simulink model "diff_drive_robot_pid_system"  (R2025a)
settings: Solver=ode15s  StartTime=0.0  StopTime=60  MaxStep=0.01  RelTol=1e-4  AbsTol=1e-6
model workspace (MAT data in the model file):
  R_robot = 0.25
  d0 = 1
  k_drag = 0.15
  m = 5
libraries: slpidlib x1
settings Model: Creator=wzy  LastModifiedBy=wzy
settings SolverCC: ZeroCrossAlgorithm=Adaptive

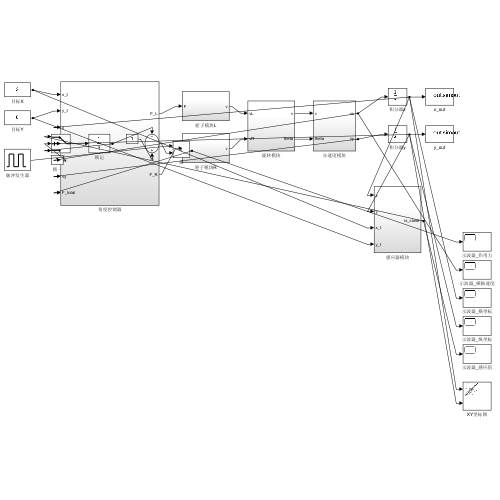
[thumbnail: Simulink's stored preview of the top-level diagram]
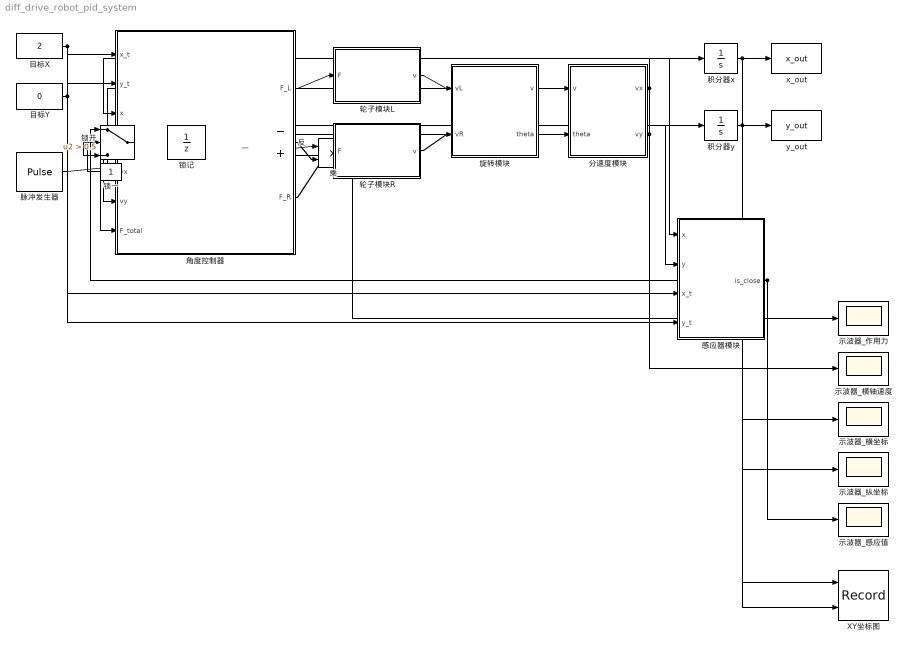
== system diff_drive_robot_pid_system ==
  XY坐标图 : Record  NumPorts=2.0  FileSettingsInternal="{\"entries\":[{\"content\":{\"excelSettings\":{\"content\":{},\"type\":\"Streamout.ExcelSettings\"},\"parquetSettings\":{\"content\":{},\"type\":\"Streamout.ParquetSettings\"}},\"type\":\"Streamout.FileSettingStorage\",\"uuid\":\"\"}],\"packageUris\":[\"http:\\/\\/schema.mathworks.com\\/mf0\\/streamout_blocks\\/R2020a\"],\"version\":\"1.0\"}"  FrameSettings=[0, 0]  Layout=[1 1]  SignalsInternal="{\"entries\":[{\"content\":{\"signals\":[{\"content\":{\"blockPath\":[],\"dimensions\":[1],\"domain\":\"\",\"lineColor\":\"#a2142f\",\"plots\":[ 1 ],\"port\":1,\"signalID\":1,\"signalName\":\"XY Graph:1\"},\"type\":\"RecordBlkView.Signal\",\"uuid\":\"\"},{\"content\":{\"blockPath\":[],\"dimensions\":[1],\"domain\":\"\",\"lineColor\":\"#139fff\",\"plots\":[ 1 ],\"port\":2,\"signalID\":2,\"signalName\":\"XY Graph:2\"},\"type\":\"RecordBlkView.Signal\",\"uuid\":\"\"}]},\"type\":\"RecordBlkView.InputSignals\",\"uuid\":\"\"}],\"packageUris\":[\"http:\\/\\/schema.mathworks.com\\/mf0\\/streamout_blocks\\/R2020a\"],\"version\":\"1.0\"}"  VisualizationBindings="{\"xyplotplugin\":{\"info\":[{\"series\":[{\"bindingParametersList\":[{\"parameter\":\"X-Axis\",\"signalID\":1,\"signalName\":\"XY Graph:1\"},{\"parameter\":\"Y-Axis\",\"signalID\":2,\"signalName\":\"XY Graph:2\"}],\"seriesID\":0}],\"subplotID\":1}]}}"  CompatibilityTag=XY
  x_out : ToWorkspace  VariableName=x_out  SampleTime=-1
  y_out : ToWorkspace  VariableName=y_out  SampleTime=-1
  一 : Constant
  乘 : Product
  分速度模块 : Subsystem
  反 : Sum  Inputs=-+
  感应器模块 : Subsystem
  旋转模块 : Subsystem
  目标X : Constant  Value=2
  目标Y : Constant  Value=0
  示波器_作用力 : Scope
  示波器_感应值 : Scope
  示波器_横坐标 : Scope
  示波器_横轴速度 : Scope
  示波器_纵坐标 : Scope
  积分器x : Integrator
  积分器y : Integrator
  脉冲发生器 : DiscretePulseGenerator  PulseType=Time based  Amplitude=0.8  PulseWidth=0.5
  角度控制器 : Subsystem
  轮子模块L : Subsystem
  轮子模块R : Subsystem
  锁一 : Constant
  锁开 : Switch  Criteria=u2 > Threshold  Threshold=0.5  SaturateOnIntegerOverflow=off  InputSameDT=off
  锁记 : UnitDelay  SampleTime=0.01  HasFrameUpgradeWarning=on
  wires:
  目标X/1 -> 角度控制器/1(x_t), 感应器模块/3(x_t)
  目标Y/1 -> 角度控制器/2(y_t), 感应器模块/4(y_t)
  角度控制器/1(F_L) -> 轮子模块L/1(F)
  角度控制器/2(F_R) -> 轮子模块R/1(F)
  轮子模块L/1(v) -> 旋转模块/1(vL)
  轮子模块R/1(v) -> 旋转模块/2(vR)
  旋转模块/1(v) -> 分速度模块/1(v)
  旋转模块/2(theta) -> 分速度模块/2(theta)
  分速度模块/1(vx) -> 积分器x/1, 角度控制器/5(vx), 示波器_横轴速度/1
  分速度模块/2(vy) -> 积分器y/1, 角度控制器/6(vy)
  积分器x/1 -> 角度控制器/3(x), 感应器模块/1(x), 示波器_横坐标/1, XY坐标图/1, x_out/1
  积分器y/1 -> 角度控制器/4(y), 感应器模块/2(y), 示波器_纵坐标/1, XY坐标图/2, y_out/1
  感应器模块/1(is_close) -> 锁开/1, 示波器_感应值/1
  锁一/1 -> 锁开/2
  锁记/1 -> 锁开/3, 反/1
  锁开/1 -> 锁记/1
  一/1 -> 反/2
  脉冲发生器/1 -> 乘/1
  反/1 -> 乘/2
  乘/1 -> 角度控制器/7(F_total), 示波器_作用力/1

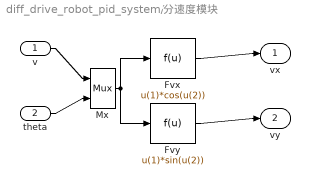
== system diff_drive_robot_pid_system/分速度模块 ==
  v : Inport
  theta : Inport  Port=2
  Fvx : Fcn  Expr=u(1)*cos(u(2))
  Fvy : Fcn  Expr=u(1)*sin(u(2))
  Mx : Mux  Inputs=2
  vx : Outport
  vy : Outport  Port=2
  wires:
  v/1 -> Mx/1
  theta/1 -> Mx/2
  Mx/1 -> Fvx/1, Fvy/1
  Fvx/1 -> vx/1
  Fvy/1 -> vy/1

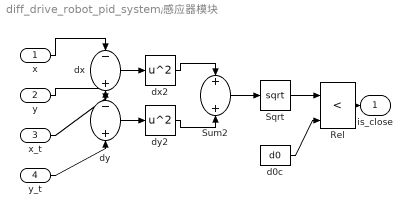
== system diff_drive_robot_pid_system/感应器模块 ==
  x : Inport
  y : Inport  Port=2
  x_t : Inport  Port=3
  y_t : Inport  Port=4
  Rel : RelationalOperator  Operator=<  OutDataTypeStr=boolean  RndMeth=Simplest  InputSameDT=off
  Sqrt : Sqrt
  Sum2 : Sum
  d0c : Constant  Value=d0
  dx : Sum  Inputs=-+
  dx2 : Math  Operator=square
  dy : Sum  Inputs=-+
  dy2 : Math  Operator=square
  is_close : Outport
  wires:
  x/1 -> dx/1
  x_t/1 -> dx/2
  y/1 -> dy/1
  y_t/1 -> dy/2
  dx/1 -> dx2/1
  dy/1 -> dy2/1
  dx2/1 -> Sum2/1
  dy2/1 -> Sum2/2
  Sum2/1 -> Sqrt/1
  Sqrt/1 -> Rel/1
  d0c/1 -> Rel/2
  Rel/1 -> is_close/1

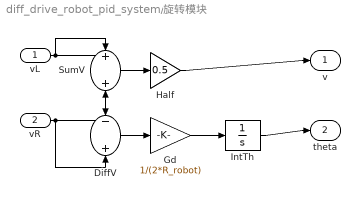
== system diff_drive_robot_pid_system/旋转模块 ==
  vL : Inport
  vR : Inport  Port=2
  DiffV : Sum  Inputs=-+
  Gd : Gain  Gain=1/(2*R_robot)
  Half : Gain  Gain=0.5
  IntTh : Integrator
  SumV : Sum
  v : Outport
  theta : Outport  Port=2
  wires:
  vL/1 -> SumV/1, DiffV/1
  vR/1 -> SumV/2, DiffV/2
  SumV/1 -> Half/1
  Half/1 -> v/1
  DiffV/1 -> Gd/1
  Gd/1 -> IntTh/1
  IntTh/1 -> theta/1

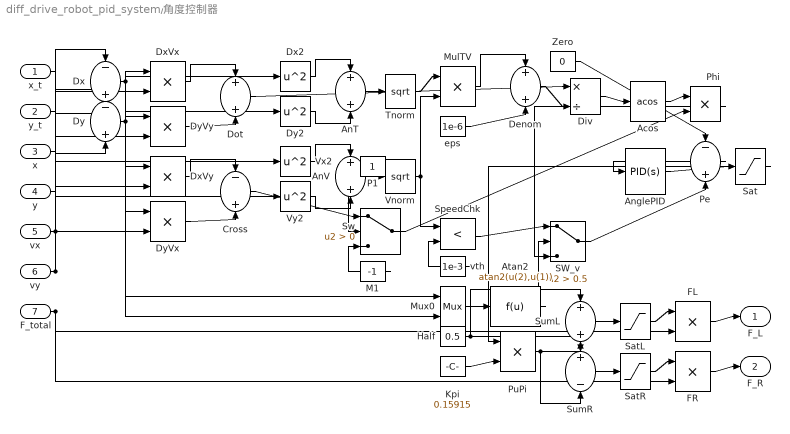
== system diff_drive_robot_pid_system/角度控制器 ==
  x_t : Inport
  y_t : Inport  Port=2
  x : Inport  Port=3
  y : Inport  Port=4
  vx : Inport  Port=5
  vy : Inport  Port=6
  F_total : Inport  Port=7
  Acos : Trigonometry  Operator=acos
  AnT : Sum
  AnV : Sum
  AnglePID : slpidlib/PID Controller  Controller=PID  Form=Parallel  TimeDomain=Continuous-time  UseExternalTs=off  SampleTime=-1  IntegratorMethod=Forward Euler  FilterMethod=Forward Euler  ControllerParametersSource=internal  P=3  I=0  UseKiTs=off  D=0  UseExternalDerivativeSource=off  N=100  UseFilter=on  TunerSelectOption=Transfer Function Based (PID Tuner App)  InitialConditionSource=internal  InitialConditionForIntegrator=0  InitialConditionForFilter=0  DifferentiatorICPrevScaledInput=0  ExternalReset=none  TrackingMode=off  Kt=1  LimitOutput=off  SatLimitsSource=internal  UpperSaturationLimit=inf  LowerSaturationLimit=-inf  LinearizeAsGain=on  AntiWindupMode=none  Kb=1  LimitIntegrator=off  UpperIntegratorSaturationLimit=inf  LowerIntegratorSaturationLimit=-inf  POutMin=[]  POutMax=[]  IOutMin=[]  IOutMax=[]  DOutMin=[]  DOutMax=[]  NOutMin=[]  NOutMax=[]  SumOutMin=[]  SumOutMax=[]  SaturationOutMin=[]  SaturationOutMax=[]  PParamMin=[]  PParamMax=[]  IParamMin=[]  IParamMax=[]  DParamMin=[]  DParamMax=[]  NParamMin=[]  NParamMax=[]  KbParamMin=[]  KbParamMax=[]  KtParamMin=[]  KtParamMax=[]  KbOutMin=[]  KbOutMax=[]  KtOutMin=[]  KtOutMax=[]  IntegratorOutMin=[]  IntegratorOutMax=[]  FilterOutMin=[]  FilterOutMax=[]  SumI1OutMin=[]  SumI1OutMax=[]  SumI2OutMin=[]  SumI2OutMax=[]  SumI3OutMin=[]  SumI3OutMax=[]  SumI4OutMin=[]  SumI4OutMax=[]  SumDOutMin=[]  SumDOutMax=[]  DifferentiatorOutMin=[]  DifferentiatorOutMax=[]  FilterDiffOutCoefMin=[]  FilterDiffOutCoefMax=[]  ReciprocalOutMin=[]  ReciprocalOutMax=[]  SumDenOutMin=[]  SumDenOutMax=[]  SumNumOutMin=[]  SumNumOutMax=[]  DivideOutMin=[]  DivideOutMax=[]  UdiffTsProdOutMin=[]  UdiffTsProdOutMax=[]  NTsProdOutMin=[]  NTsProdOutMax=[]  UintegralTsProdOutMin=[]  UintegralTsProdOutMax=[]  UngainTsProdOutMin=[]  UngainTsProdOutMax=[]  ClampingZeroOutDataTypeStr=Inherit: Inherit via back propagation  ClampingZeroOutMin=[]  ClampingZeroOutMax=[]  FilterDenConstantOutDataTypeStr=Inherit: Inherit via back propagation  FilterDenConstantOutMin=[]  FilterDenConstantOutMax=[]  PCopyOutDataTypeStr=Inherit: Inherit via back propagation  PCopyOutMin=[]  PCopyOutMax=[]  NCopyOutDataTypeStr=Inherit: Inherit via back propagation  NCopyOutMin=[]  NCopyOutMax=[]  IntegratorContinuousStateAttributes=''  IntegratorStateMustResolveToSignalObject=off  IntegratorRTWStateStorageClass=Auto  FilterContinuousStateAttributes=''  FilterStateMustResolveToSignalObject=off  FilterRTWStateStorageClass=Auto  ParallelPVariant=InternalParameters  IdealPVariant=Disabled  IVariant=InternalParameters  DVariant=InternalParameters  IntegratorVariant=Continuous  SatVariant=Disabled  AWVariant=Passthrough  PCopyVariant=Disabled  TRVariant=Disabled  FdbkBlocksVariant=Forward  IdealPFdbkVariant=Disabled  SatFdbkVariant=Disabled  DerivativeFilterVariant=ContFilter  NVariant=InternalParameters  NCopyVariant=Disabled  FilterICVariant=InternalICsFilter  IntegratorICVariant=InternalICs  ExternalResetVariant=Disabled  TRSumVariant=Passthrough  SumFdbkVariant=Disabled  SumVariant=Sum_PID  TsampFilterVariant=InternalTs  TsampNgainVariant=Passthrough  TsampIntegralVariant=Disabled_SignalSpec  ExternalSaturationOutDataTypeStr=Inherit: Same as second input  DerivativeSourceVariant=ErrorSignal  PreIntVariant=InternalPreInt
  Atan2 : Fcn  Expr=atan2(u(2),u(1))
  Cross : Sum  Inputs=-+
  Denom : Sum
  Div : Product  Inputs=*/
  Dot : Sum
  Dx : Sum  Inputs=-+
  Dx2 : Math  Operator=square
  DxVx : Product
  DxVy : Product
  Dy : Sum  Inputs=-+
  Dy2 : Math  Operator=square
  DyVx : Product
  DyVy : Product
  FL : Product
  FR : Product
  Half : Constant  Value=0.5
  Kpi : Constant  Value=0.15915
  M1 : Constant  Value=-1
  MulTV : Product
  Mux0 : Mux  Inputs=2
  P1 : Constant
  Pe : Sum  Inputs=-+
  Phi : Product
  PuPi : Product
  SW_v : Switch  Criteria=u2 > Threshold  Threshold=0.5  ZeroCross=off  SaturateOnIntegerOverflow=off  InputSameDT=off
  Sat : Saturate  UpperLimit=3.1416  LowerLimit=-3.1416  ZeroCross=off
  SatL : Saturate  UpperLimit=1  LowerLimit=-1  ZeroCross=off
  SatR : Saturate  UpperLimit=1  LowerLimit=-1  ZeroCross=off
  SpeedChk : RelationalOperator  Operator=<  OutDataTypeStr=boolean  ZeroCross=off  RndMeth=Simplest  InputSameDT=off
  SumL : Sum
  SumR : Sum  Inputs=+-
  Sw : Switch  Criteria=u2 > Threshold  ZeroCross=off  SaturateOnIntegerOverflow=off  InputSameDT=off
  Tnorm : Sqrt
  Vnorm : Sqrt
  Vx2 : Math  Operator=square
  Vy2 : Math  Operator=square
  Zero : Constant  Value=0
  eps : Constant  Value=1e-6
  vth : Constant  Value=1e-3
  F_L : Outport
  F_R : Outport  Port=2
  wires:
  x/1 -> Dx/1
  x_t/1 -> Dx/2
  y/1 -> Dy/1
  y_t/1 -> Dy/2
  Dx/1 -> DxVx/1, DxVy/1, Dx2/1, Mux0/1
  vx/1 -> DxVx/2, DyVx/2, Vx2/1
  Dy/1 -> DyVy/1, DyVx/1, Dy2/1, Mux0/2
  vy/1 -> DyVy/2, DxVy/2, Vy2/1
  DxVx/1 -> Dot/1
  DyVy/1 -> Dot/2
  DxVy/1 -> Cross/1
  DyVx/1 -> Cross/2
  Dx2/1 -> AnT/1
  Dy2/1 -> AnT/2
  AnT/1 -> Tnorm/1
  Vx2/1 -> AnV/1
  Vy2/1 -> AnV/2
  AnV/1 -> Vnorm/1
  Tnorm/1 -> MulTV/1
  Vnorm/1 -> MulTV/2, SpeedChk/1
  MulTV/1 -> Denom/1
  eps/1 -> Denom/2
  Denom/1 -> Div/2
  Dot/1 -> Div/1
  Div/1 -> Acos/1
  Cross/1 -> Sw/1
  P1/1 -> Sw/2
  M1/1 -> Sw/3
  Acos/1 -> Phi/1
  Sw/1 -> Phi/2
  vth/1 -> SpeedChk/2
  Mux0/1 -> Atan2/1
  SpeedChk/1 -> SW_v/1
  Atan2/1 -> SW_v/2
  Phi/1 -> SW_v/3
  Zero/1 -> Pe/1
  SW_v/1 -> Pe/2
  Pe/1 -> AnglePID/1
  AnglePID/1 -> Sat/1
  Sat/1 -> PuPi/1
  Kpi/1 -> PuPi/2
  Half/1 -> SumL/1, SumR/1
  PuPi/1 -> SumL/2, SumR/2
  SumL/1 -> SatL/1
  SumR/1 -> SatR/1
  SatL/1 -> FL/1
  F_total/1 -> FL/2, FR/2
  SatR/1 -> FR/1
  FL/1 -> F_L/1
  FR/1 -> F_R/1

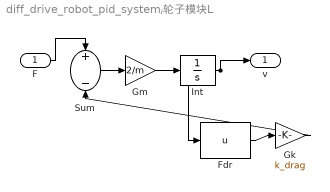
== system diff_drive_robot_pid_system/轮子模块L ==
  F : Inport
  Fdr : Fcn  Expr=u
  Gk : Gain  Gain=k_drag
  Gm : Gain  Gain=2/m
  Int : Integrator
  Sum : Sum  Inputs=+-
  v : Outport
  wires:
  F/1 -> Sum/1
  Sum/1 -> Gm/1
  Gm/1 -> Int/1
  Int/1 -> v/1, Fdr/1
  Fdr/1 -> Gk/1
  Gk/1 -> Sum/2

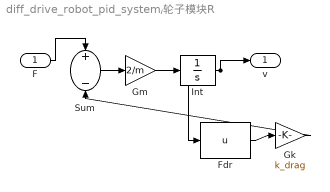
== system diff_drive_robot_pid_system/轮子模块R ==
  F : Inport
  Fdr : Fcn  Expr=u
  Gk : Gain  Gain=k_drag
  Gm : Gain  Gain=2/m
  Int : Integrator
  Sum : Sum  Inputs=+-
  v : Outport
  wires:
  F/1 -> Sum/1
  Sum/1 -> Gm/1
  Gm/1 -> Int/1
  Int/1 -> v/1, Fdr/1
  Fdr/1 -> Gk/1
  Gk/1 -> Sum/2
